simulink model "satr"  (R2017a)
settings: Solver=VariableStepAuto  StartTime=0.0  StopTime=inf  RelTol=1e-3
libraries: dspsrcs4 x1
settings Model: Creator=ilyas  LastModifiedBy=ilyas

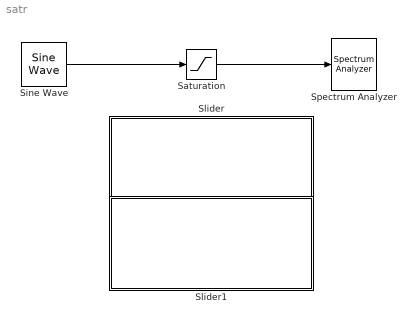
== system satr ==
  Saturation : Saturate  UpperLimit=9.565217391304  LowerLimit=5.2173913043478
  Sine Wave : dspsrcs4/Sine Wave  Amplitude=1  Frequency=100  Phase=0  SampleMode=Discrete  OutComplex=Real  CompMethod=Trigonometric fcn  TableSize=Speed  SampleTime=1/11025  SamplesPerFrame=1024  ResetState=Restart at time zero  OutputFrames=off  dataType=double  wordLen=16  udDataType=sfix(16)  fracBitsMode=Best precision  numFracBits=15  OutDataTypeStr=double  LastOutDataTypeStr=double
  Slider : Subsystem  DialogController=hmiCreateDDGDialog  IsWebBlock=on  mask(MWDashboardBlock){webBlockId=40fb5c0a-deff-44ca-9fc8-20ff7acc1f2b, webBlockType=slider, ShowInLibBrowser=on, ShowInitialText=on, HMISrcModelName=untitled}
      mask prompts: webBlockId "WebBlock Id"; webBlockType "WebBlock Type"; HMISrcModelName "Source Model"
      mask help: SimulinkHMI:dialogs:SliderDialogDesc
      mask Help: helpview([docroot '/mapfiles/simulink.map'], 'hmi_slider')
      mask Display:
      | if strcmp(get_param(bdroot(gcb),'BlockDiagramType'), 'library')
      |     image([(matlabroot) '/toolbox/simulink/hmi/icons/Slider.png']);
      | end
  Slider1 : Subsystem  DialogController=hmiCreateDDGDialog  IsWebBlock=on  mask(MWDashboardBlock){webBlockId=48527fc2-e127-4412-ba00-1c4c26db83f7, webBlockType=slider, ShowInLibBrowser=on, ShowInitialText=on, HMISrcModelName=untitled}
      mask prompts: webBlockId "WebBlock Id"; webBlockType "WebBlock Type"; HMISrcModelName "Source Model"
      mask help: SimulinkHMI:dialogs:SliderDialogDesc
      mask Help: helpview([docroot '/mapfiles/simulink.map'], 'hmi_slider')
      mask Display:
      | if strcmp(get_param(bdroot(gcb),'BlockDiagramType'), 'library')
      |     image([(matlabroot) '/toolbox/simulink/hmi/icons/Slider.png']);
      | end
  Spectrum Analyzer : SpectrumAnalyzer
  wires:
  Sine Wave/1 -> Saturation/1
  Saturation/1 -> Spectrum Analyzer/1

== system satr/Slider ==

== system satr/Slider1 ==
